simulink model "untitled"  (R2018b)
settings: Solver=VariableStepAuto  StartTime=0.0  StopTime=10.0  RelTol=1e-3
libraries: dsparch4 x1
settings Model: Creator=nhat  LastModifiedBy=nhat

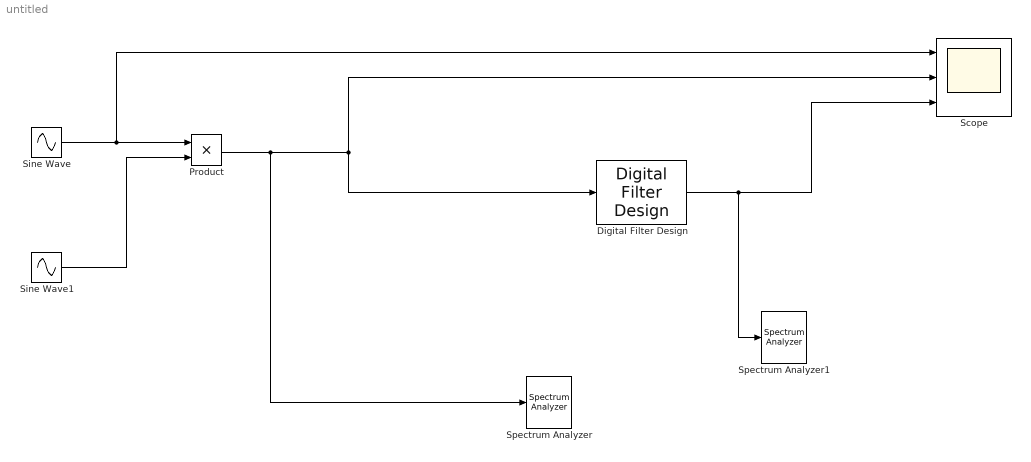
== system untitled ==
  Digital Filter Design : dsparch4/Digital Filter Design  mwdsp_browser_bugfix_var=off
  Product : Product
  Scope : Scope  NumInputPorts=3
  Sine Wave : Sin  Frequency=1000*2*pi  SampleTime=1/20000
  Sine Wave1 : Sin  Frequency=5000*pi*2  SampleTime=1/20000
  Spectrum Analyzer : SpectrumAnalyzer
  Spectrum Analyzer1 : SpectrumAnalyzer
  wires:
  Sine Wave1/1 -> Product/2
  Sine Wave/1 -> Scope/1, Product/1
  Product/1 -> Spectrum Analyzer/1, Digital Filter Design/1, Scope/2
  Digital Filter Design/1 -> Spectrum Analyzer1/1, Scope/3
